simulink model "VehicleSteering_sim_Int"  (R2020a)
settings: Solver=VariableStepAuto  StartTime=0.0  StopTime=10.0  RelTol=1e-3
values from neighbouring files (symbols this model uses):
  A = [0 v0;0 0]    [Example_VehicleSteering_Ackermann.m]    (also in Example_VehicleSteering_Integral_action.m = Ag; Example_VehicleSteering_SS_control.m)
  B = [a*v0/b v0/b]'    [Example_VehicleSteering_Ackermann.m]    (also in Example_VehicleSteering_Integral_action.m = Bg; Example_VehicleSteering_SS_control.m)
  C = eye(2)    [Example_VehicleSteering_Ackermann.m]    (also in Example_VehicleSteering_Integral_action.m = eye(3); Example_VehicleSteering_SS_control.m)
  D = [0 0]'    [Example_VehicleSteering_Ackermann.m]    (also in Example_VehicleSteering_Integral_action.m = [0 0 0]'; Example_VehicleSteering_SS_control.m)
undefined symbols (not defined in the file or in its folder): Ku
settings Model: Creator=jofr  LastModifiedBy=rodralez
settings DataIOCC: ReturnWorkspaceOutputs=off
settings DebuggingCC: ArithmeticOperatorsInVariantConditions=warning
settings SFSimCC: SimUseLocalCustomCode=off  CustomCodeUndefinedFunction=UseInterfaceOnly
settings RTWCC: RTWUseLocalCustomCode=off

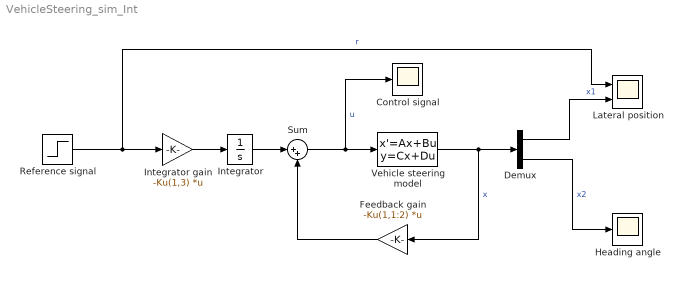
== system VehicleSteering_sim_Int ==
  Control signal : Scope
  Demux : Demux  Outputs=2
  Feedback gain : Gain  Gain=-Ku(1,1:2)  Multiplication=Matrix(K*u)
  Heading angle : Scope
  Integrator : Integrator
  Integrator gain : Gain  Gain=-Ku(1,3)  Multiplication=Matrix(K*u)
  Lateral position : Scope  NumInputPorts=2
  "Reference signal " : Step  SampleTime=0
  Sum : Sum  Inputs=|++
  Vehicle steering model : StateSpace  A=A  B=B  C=C  D=D  InitialCondition=0
  wires:
  Vehicle steering model/1 -> Demux/1, Feedback gain/1  "x"
  Sum/1 -> Control signal/1, Vehicle steering model/1  "u"
  Feedback gain/1 -> Sum/2
  Demux/2 -> Heading angle/1  "x2"
  "Reference signal "/1 -> Integrator gain/1, Lateral position/1  "r"
  Demux/1 -> Lateral position/2  "x1"
  Integrator gain/1 -> Integrator/1
  Integrator/1 -> Sum/1
